simulink model "SF5_2_4_jc_0531_2"  (R2016b)
settings: Solver=VariableStepAuto  StartTime=0.0  StopTime=10.0  RelTol=1e-3
settings Model: Creator=amyyang  LastModifiedBy=amyyang

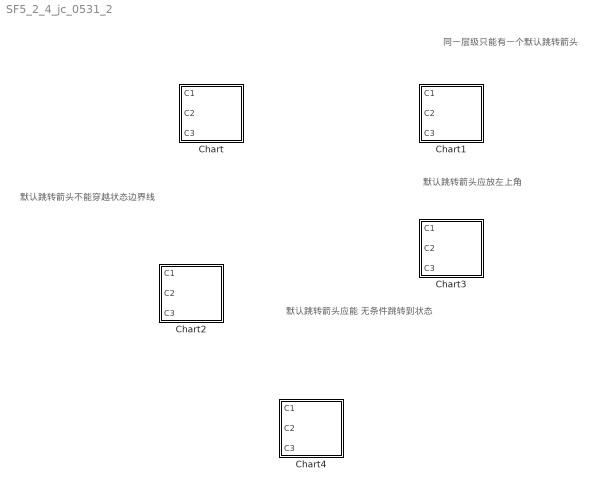
== system SF5_2_4_jc_0531_2 ==
  note: 默认跳转箭头应能
      | 无条件跳转到状态
  note: 默认跳转箭头不能穿越状态边界线
  note: 默认跳转箭头应放左上角
  note: 同一层级只能有一个默认跳转箭头
  Chart : Stateflow chart  TreatAsAtomicUnit=on
  Chart1 : Stateflow chart  TreatAsAtomicUnit=on
  Chart2 : Stateflow chart  TreatAsAtomicUnit=on
  Chart3 : Stateflow chart  TreatAsAtomicUnit=on
  Chart4 : Stateflow chart  TreatAsAtomicUnit=on

== stateflow chart SF5_2_4_jc_0531_2/Chart1 ==
  note: 同一层级只能有一个默认跳转箭头
  state A1
    state AA
    state BB
    (default) -> AA [order 1]
    BB -> AA : [C2]
    AA -> BB : [C3]
    (default) -> BB [order 2]
  state B1
  (default) -> A1
  A1 -> B1 : [C4]
  B1 -> A1 : [C5]
  data: C1 input; C2 input; C3 input

== stateflow chart SF5_2_4_jc_0531_2/Chart2 ==
  note: 默认跳转箭头不能穿越状态边界线
  state A
    state AA
    state BB
    (junction 10) -> AA [order 1] : [C1]
    (junction 10) -> (junction 13) [order 2]
    BB -> AA : [C2]
    AA -> BB : [C3]
    (junction 13) -> BB
  state B
  (default) -> A [order 1]
  (default) -> (junction 10) [order 2]
  A -> B : [C4]
  B -> A : [C5]
  data: C1 input; C2 input; C3 input

== stateflow chart SF5_2_4_jc_0531_2/Chart ==
  state A
    state AA
    state BB
    (default) -> (junction 10)
    (junction 10) -> AA [order 1] : [C1]
    (junction 10) -> (junction 13) [order 2]
    BB -> AA : [C2]
    AA -> BB : [C3]
    (junction 13) -> BB
  state B
  (default) -> A
  A -> B : [C4]
  B -> A : [C5]
  data: C1 input; C2 input; C3 input

== stateflow chart SF5_2_4_jc_0531_2/Chart3 ==
  note: 默认跳转箭头应放左上角
  state A
    state AA
    state BB
    AA -> BB : [C3]
    BB -> AA : [C2]
    (default) -> BB
  state B
  A -> B : [C4]
  (default) -> A
  B -> A : [C5]
  data: C1 input; C2 input; C3 input

== stateflow chart SF5_2_4_jc_0531_2/Chart4 ==
  state A
    state AA
    state BB
    (default) -> (junction 10)
    (junction 10) -> AA [order 1] : [C1]
    (junction 10) -> (junction 13) [order 2]
    BB -> AA : [C2]
    AA -> BB : [C3]
    (junction 13) -> BB : [C6]
  state B
  (default) -> A
  A -> B : [C4]
  B -> A : [C5]
  data: C1 input; C2 input; C3 input
